simulink model "idealConverter_2"  (R2018a)
settings: Solver=VariableStepDiscrete  StartTime=0.0  StopTime=0.002  RelTol=1e-3
libraries: powerlib x17, powerlib_meascontrol x1
settings Model: Creator=ekoma  LastModifiedBy=mertelmas

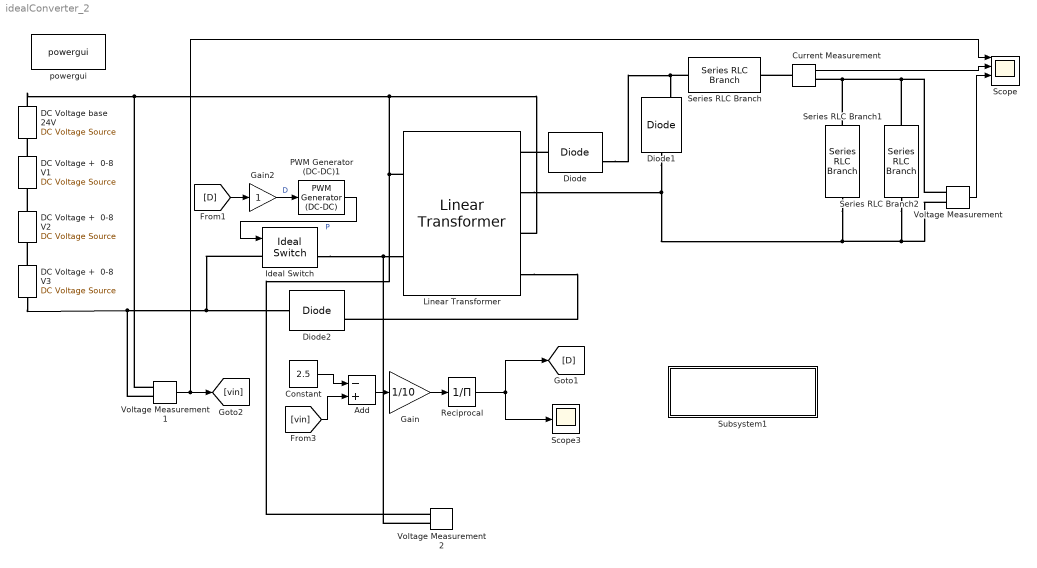
== system idealConverter_2 ==
  Add : Sum  Inputs=-+
  Constant : Constant  Value=2.5
  Current Measurement : powerlib/Measurements/Current Measurement  PhasorSimulation=off  OutputType=Complex  PSBequivalent=0
  DC Voltage +  0-8 V1 : powerlib/Electrical Sources/DC Voltage Source  Amplitude=8  Measurements=None
  DC Voltage +  0-8 V2 : powerlib/Electrical Sources/DC Voltage Source  Amplitude=8  Measurements=None
  DC Voltage +  0-8 V3 : powerlib/Electrical Sources/DC Voltage Source  Amplitude=8  Measurements=None
  DC Voltage base 24V : powerlib/Electrical Sources/DC Voltage Source  Amplitude=24  Measurements=None
  Diode : powerlib/Power Electronics/Diode  Ron=0.001  Lon=0  Vf=0.8  IC=0  UseSnubber=0  Rs=500  Cs=250e-9  Measurements=on
  Diode1 : powerlib/Power Electronics/Diode  Ron=0.001  Lon=0  Vf=0.8  IC=0  UseSnubber=0  Rs=500  Cs=250e-9  Measurements=on
  Diode2 : powerlib/Power Electronics/Diode  Ron=0.001  Lon=0  Vf=0.8  IC=0  UseSnubber=0  Rs=500  Cs=250e-9  Measurements=on
  Gain : Gain  Gain=1/10
  Gain2 : Gain
  Ideal Switch : powerlib/Power Electronics/Ideal Switch  Ron=0.001  Lon=0  IC=0  Rs=1e5  Cs=inf  Measurements=on
  Linear Transformer : powerlib/Elements/Linear Transformer  UNITS=SI  NominalPower=[ 40 64000 ]  winding1=[50 0.000001 0.0000001]  winding2=[50 0.0000001 0.000001]  ThreeWindings=on  winding3=[50 0.00000001 0.00001]  RmLm=[1.0805e+06 2866]  Measurements=None  DataType=on
  PWM Generator (DC-DC)1 : powerlib_meascontrol/Pulse & Signal Generators/PWM Generator (DC-DC)  Fsw=32000  Ts=0
  Reciprocal : Product  Inputs=/
  Scope : Scope  NumInputPorts=4
  Scope3 : Scope
  Series RLC Branch : powerlib/Elements/Series RLC Branch  LConnTagsString=__new0  RConnTagsString=__new0  BranchType=L  Resistance=1  Inductance=220e-6  SetiL0=off  InitialCurrent=0  Capacitance=1e-6  Setx0=off  InitialVoltage=0  Measurements=None
  Series RLC Branch1 : powerlib/Elements/Series RLC Branch  LConnTagsString=__new0  RConnTagsString=__new0  BranchType=C  Resistance=1  Inductance=1e-3  SetiL0=off  InitialCurrent=0  Capacitance=47e-6  Setx0=off  InitialVoltage=0  Measurements=None
  Series RLC Branch2 : powerlib/Elements/Series RLC Branch  LConnTagsString=__new0  RConnTagsString=__new0  BranchType=R  Resistance=2.5  Inductance=1e-3  SetiL0=off  InitialCurrent=0  Capacitance=1e-6  Setx0=off  InitialVoltage=0  Measurements=None
  Subsystem1 : Subsystem
      settings: OpenFcn=open_system('power_new_palette')
      mask Display: disp(sprintf('Open Simscape Power Systems\n(Specialized Technology)\nPalette Library'));
  Voltage Measurement : powerlib/Measurements/Voltage Measurement  PhasorSimulation=off  OutputType=Complex  PSBequivalent=0
  Voltage Measurement1 : powerlib/Measurements/Voltage Measurement  PhasorSimulation=off  OutputType=Complex  PSBequivalent=0
  Voltage Measurement2 : powerlib/Measurements/Voltage Measurement  PhasorSimulation=off  OutputType=Complex  PSBequivalent=0
  powergui : powerlib/powergui  Priority=1  SimulationMode=Discrete  SampleTime=1e-7  frequency=60  Iterations=50  frequencyindice=0  Pbase=100e6  ErrMax=1e-4  UnitsV=kV  UnitsW=MW  buscounter=0  FunctionMessages=off  echomessages=off  EnableUseOfTLC=off  CurrentSourceSwitches=off  DisableSnubberDevices=off  DisableRonSwitches=off  DisableVfSwitches=off  DisplayEquations=off  SolverType=Tustin/Backward Euler (TBE)  Interpol=off  ExternalGateDelay=off  methode=off  Ts=100  x0status=blocks  SPID=on  SwTol=0  HookPort=off  RestoreLinks=warning  ResistiveCurrentMeasurement=off  Frange=[0:2:500]  Ylog=off  Xlog=on  ShowGrid=off  save=off  variable=ZData  structure=0  ZoomFFT=off  StartTime=0.0  cycles=1  DisplayStyle=1  fundamental=60  FreqAxis=off  MaxFrequency=1000  frequencyindicesteady=1  RmsSteady=1  display=off
  wires:
  Current Measurement/1 -> Scope/2
  Voltage Measurement/1 -> Scope/3
  Reciprocal/1 -> [D], Scope3/1
  Gain2/1 -> PWM Generator (DC-DC)1/1  "D"
  Gain/1 -> Reciprocal/1
  [D] -> Gain2/1
  Voltage Measurement1/1 -> [vin], Scope/1
  PWM Generator (DC-DC)1/1 -> Ideal Switch/1  "P"
  [vin] -> Add/2
  Constant/1 -> Add/1
  Add/1 -> Gain/1
  connections:
  Diode/LConn1 -- Linear Transformer/RConn1
  Diode/RConn1 -- Series RLC Branch/LConn1 -- Diode1/RConn1
  Current Measurement/LConn1 -- Series RLC Branch/RConn1
  Series RLC Branch2/LConn1 -- Voltage Measurement/LConn1 -- Series RLC Branch1/LConn1 -- Current Measurement/RConn1
  Linear Transformer/LConn1 -- Voltage Measurement1/LConn1 -- DC Voltage base 24V/RConn1 -- Linear Transformer/RConn3 -- Voltage Measurement2/LConn1
  Series RLC Branch2/RConn1 -- Voltage Measurement/LConn2 -- Linear Transformer/RConn2 -- Diode1/LConn1 -- Series RLC Branch1/RConn1
  Linear Transformer/RConn4 -- Diode2/RConn1
  Ideal Switch/RConn1 -- Voltage Measurement2/LConn2 -- Linear Transformer/LConn2
  Ideal Switch/LConn1 -- Voltage Measurement1/LConn2 -- DC Voltage +  0-8 V3/LConn1 -- Diode2/LConn1
  DC Voltage +  0-8 V1/RConn1 -- DC Voltage base 24V/LConn1
  DC Voltage +  0-8 V2/RConn1 -- DC Voltage +  0-8 V1/LConn1
  DC Voltage +  0-8 V3/RConn1 -- DC Voltage +  0-8 V2/LConn1

== system idealConverter_2/Subsystem1 ==
